simulink model "teste_controlador"  (R2018b)
settings: Solver=ode4  StartTime=0.0  StopTime=0.1  FixedStep=0.0001  RelTol=1e-3
InitFcn:
  | J = 0.916e-6;
  | B = 0.66e-6;
  | a0 = 0.738e-12;
  | a1 = 0.198e-10;
libraries: simulink x1
settings Model: Creator=easylab  LastModifiedBy=easylab

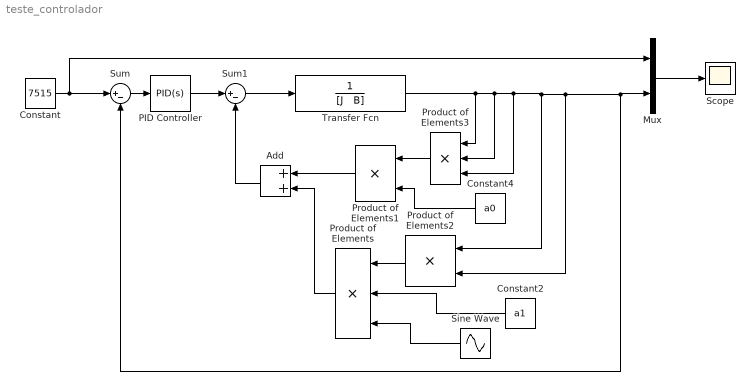
== system teste_controlador ==
  Add : Sum
  Constant : Constant  Value=7515
  Constant2 : Constant  Value=a1
  Constant4 : Constant  Value=a0
  Mux : Mux  Inputs=2
  PID Controller : simulink/Continuous/PID Controller  Controller=PID  Form=Parallel  TimeDomain=Continuous-time  SampleTime=-1  IntegratorMethod=Forward Euler  FilterMethod=Forward Euler  ControllerParametersSource=internal  P=0.0001  I=0.1  D=0  UseFilter=on  N=100  TunerSelectOption=Transfer Function Based (PID Tuner App)  InitialConditionSource=internal  InitialConditionForIntegrator=0  InitialConditionForFilter=0  DifferentiatorICPrevScaledInput=0  ExternalReset=none  TrackingMode=off  Kt=1  LimitOutput=off  UpperSaturationLimit=inf  LowerSaturationLimit=-inf  LinearizeAsGain=on  AntiWindupMode=none  Kb=1  POutMin=[]  POutMax=[]  IOutMin=[]  IOutMax=[]  DOutMin=[]  DOutMax=[]  NOutMin=[]  NOutMax=[]  SumOutMin=[]  SumOutMax=[]  SaturationOutMin=[]  SaturationOutMax=[]  PParamMin=[]  PParamMax=[]  IParamMin=[]  IParamMax=[]  DParamMin=[]  DParamMax=[]  NParamMin=[]  NParamMax=[]  KbParamMin=[]  KbParamMax=[]  KtParamMin=[]  KtParamMax=[]  KbOutMin=[]  KbOutMax=[]  KtOutMin=[]  KtOutMax=[]  IntegratorOutMin=[]  IntegratorOutMax=[]  FilterOutMin=[]  FilterOutMax=[]  SumI1OutMin=[]  SumI1OutMax=[]  SumI2OutMin=[]  SumI2OutMax=[]  SumI3OutMin=[]  SumI3OutMax=[]  SumI4OutMin=[]  SumI4OutMax=[]  SumDOutMin=[]  SumDOutMax=[]  DifferentiatorOutMin=[]  DifferentiatorOutMax=[]  FilterDiffOutCoefMin=[]  FilterDiffOutCoefMax=[]  ReciprocalOutMin=[]  ReciprocalOutMax=[]  SumDenOutMin=[]  SumDenOutMax=[]  SumNumOutMin=[]  SumNumOutMax=[]  DivideOutMin=[]  DivideOutMax=[]  IntegratorContinuousStateAttributes=''  IntegratorStateMustResolveToSignalObject=off  IntegratorRTWStateStorageClass=Auto  FilterContinuousStateAttributes=''  FilterStateMustResolveToSignalObject=off  FilterRTWStateStorageClass=Auto  ParallelPVariant=InternalParameters  IdealPVariant=Disabled  IVariant=InternalParameters  DVariant=InternalParameters  IntegratorVariant=Continuous  SatVariant=Disabled  AWVariant=Passthrough  PCopyVariant=Disabled  TRVariant=Disabled  FdbkBlocksVariant=Forward  IdealPFdbkVariant=Disabled  SatFdbkVariant=Disabled  DerivativeFilterVariant=ContFilter  NVariant=InternalParameters  NCopyVariant=Disabled  FilterICVariant=InternalICsFilter  IntegratorICVariant=InternalICs  ExternalResetVariant=Disabled  TRSumVariant=Passthrough  SumFdbkVariant=Disabled  SumVariant=Sum_PID
  Product of Elements : Product  Inputs=3
  Product of Elements1 : Product
  Product of Elements2 : Product
  Product of Elements3 : Product  Inputs=3
  Scope : Scope
  Sine Wave : Sin  Amplitude=92  Bias=100  Frequency=2*pi*(1/0.67)  SampleTime=0
  Sum : Sum  Inputs=|+-
  Sum1 : Sum  Inputs=|+-
  Transfer Fcn : TransferFcn  Denominator="[J   B]"
  wires:
  Sum1/1 -> Transfer Fcn/1
  Product of Elements2/1 -> Product of Elements/1
  Constant2/1 -> Product of Elements/2
  Sine Wave/1 -> Product of Elements/3
  Constant4/1 -> Product of Elements1/2
  Product of Elements1/1 -> Add/1
  Product of Elements/1 -> Add/2
  Add/1 -> Sum1/2
  Transfer Fcn/1 -> Product of Elements3/1, Product of Elements3/2, Product of Elements3/3, Product of Elements2/1, Product of Elements2/2, Sum/2, Mux/2
  Mux/1 -> Scope/1
  Product of Elements3/1 -> Product of Elements1/1
  Sum/1 -> PID Controller/1
  PID Controller/1 -> Sum1/1
  Constant/1 -> Mux/1, Sum/1
